simulink model "floating_2_bodies_simple"  (Simulink 6.3)
settings: Solver=ode15s  StartTime=0.0  StopTime=inf  FixedStep=0.02  RelTol=1e-3
PreLoadFcn:
  | Body_Shv_Double_066
InitFcn:
  | mech_slider_open_ShV(gcs);
libraries: mblibv1 x12
settings Model: LastModifiedBy=Alex
settings SimMechanicsCC: VisOnUpdateDiagram=on  VisDuringSimulation=on

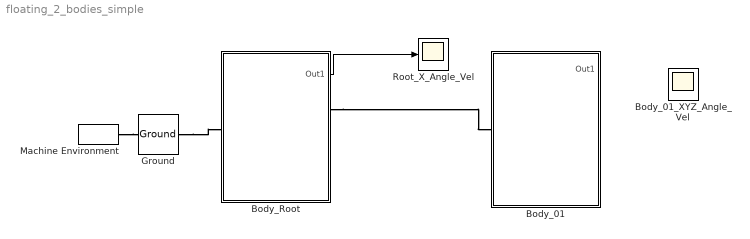
== system floating_2_bodies_simple ==
  Body_01 : Subsystem
  Body_01_XYZ_Angle_Vel : Scope
      settings: TimeRange=600  YMin=-25  YMax=2.5
  Body_Root : Subsystem
  Ground : mblibv1/Bodies/Ground  LeftPortType=env  RightPortType=workingframe  PhysicalDomain=Mechanical  DialogClass=GroundBlock  CoordPosition=[0 0 0]  CoordPositionUnits=m  StateVectorMgrId=-1  MachineId=[1 1]  ShowEnvPort=on
  Machine Environment : mblibv1/Bodies/Machine Environment  Tag=Factory ground  DialogController=MECH.DialogSource  PortType=env  PhysicalDomain=Mechanical  DialogTemplateClass=MECH.MachineEnvironment  SyncWhenCopied=off  Gravity=[0 0 0]  GravityUnits=m/s^2  GravityAsSignal=off  Dimensionality=Auto-detect  AnalysisType=Forward dynamics  LinearAssemblyTolerance=1e-3  LinearAssemblyToleranceUnits=m  AngularAssemblyTolerance=1e-3  AngularAssemblyToleranceUnits=rad  ConstraintSolverType=Stabilizing  ConstraintRelTolerance=1e-4  ConstraintAbsTolerance=1e-4  UseRobustSingularityHandling=off  StatePerturbationType=Fixed  PerturbationSize=1e-5  VisualizeMachine=on
  Root_X_Angle_Vel : Scope
      settings: TimeRange=600  YMin=-125  YMax=100
  wires:
  Body_Root/1(Out1) -> Root_X_Angle_Vel/1
  ? -> Body_01_XYZ_Angle_Vel/1
  connections:
  Machine Environment/RConn1 -- Ground/LConn1
  Ground/RConn1 -- Body_Root/LConn1
  Body_Root/RConn1 -- Body_01/LConn1

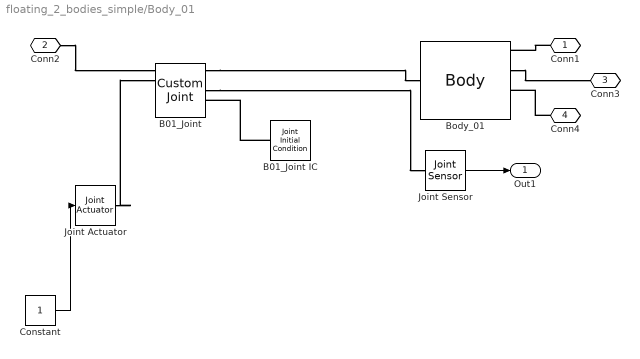
== system floating_2_bodies_simple/Body_01 ==
  B01_Joint : mblibv1/Joints/Custom Joint  PhysicalDomain=mechanical  SubClassName=custom_joint  LeftPortType=blob  RightPortType=blob  LConnTagsString=__newl0|SA1|SA2|SA3|SA4  RConnTagsString=__newr0|SA1|SA2|SA3|SA4  NumSAPorts=8  CutJoint=off  MarkAsCut=off  Primitives=revolute_revolute_revolute  PrimitiveProps=R3$WORLD$[0 0 1]$revolute#R1$WORLD$[1 0 0]$revolute#R2$WORLD$[0 1 0]$revolute  DialogClass=JointBlock
  B01_Joint IC : mblibv1/Sensors &  Actuators/Joint Initial Condition  Orientation=left  PhysicalDomain=mechanical  DialogClass=InitialConditionBlock  InitialConditions=P1$false$0$m$rad$0$m/s$rad/s#P2$false$0$m$rad$0$m/s$rad/s#P3$false$0$m$rad$0$m/s$rad/s#R1$false$0$m$rad$0$m/s$rad/s#R2$false$0$m$rad$0$m/s$rad/s#R3$false$30$m$deg$0$m/s$rad/s#S$false$0$m$rad$0$m/s$rad/s
  Body_01 : mblibv1/Bodies/Body  PhysicalDomain=mechanical  SubClassName=Unknown  LeftPortType=workingframe  RightPortType=workingframe  LConnTagsString=CS1  RConnTagsString=CS2|CS3|CS4|CS5  DialogClass=MechanicalBodyBlock  Mass=1  MassUnits=kg  InertiaUnits=kg*m^2  Inertia=[ 1/12 0 0; 0 .001 0; 0 0 1/12]  Shape=Cylinder  ShapeDims=[1 1]  ShapeUnits=m  ShapeUse=false  Density=1  DensityUnits=kg/m^3  DensityUse=false  CG=Left$CG$[0 -Body_Size 0]$CS1$CS1$m$[0 0 0]$Euler X-Y-Z$deg$WORLD$false  WorkingFrames=Left$CS1$[0 0 0]$ADJOINING$ADJOINING$m$[0 0 0]$Euler X-Y-Z$deg$WORLD$true#Right$CS2$[0 -Body_Size 0]$CG$CG$m$[0 0 0]$Euler X-Y-Z$deg$WORLD$true#Right$CS3$[-0.5*Body_Size -Body_Size 0]$CG$CG$m$[0 0 0]$Euler X-Y-Z$deg$WORLD$true#Right$CS4$[0.5*Body_Size -Body_Size 0]$CG$CG$m$[0 0 0]$Euler X-Y-Z$deg$WORLD$true#Right$CS5$[0 -Body_Size -0.2*Body_Size]$CG$CG$m$[0 0 0]$Euler X-Y-Z$deg$WORLD$true
  Constant : Constant
  Joint Actuator : mblibv1/Sensors &  Actuators/Joint Actuator  PhysicalDomain=Mechanical  PortType=blob  ActuationStyle=Force  AngleUnits=deg  ArcVelocityUnits=deg/s  ArcAccelerationUnits=deg/s^2  CoordPositionUnits=m  VelocityUnits=m/s  AccelerationUnits=m/s^2  ForceUnits=N  TorqueUnits=N-m  ActiveIO=on  Width=1  DialogClass=MechanicalActuatorBlock  Primitive=R1  ReferenceFrame=Absolute (INERTIAL)
  Joint Sensor : mblibv1/Sensors &  Actuators/Joint Sensor  PhysicalDomain=Mechanical  PortType=blob  Muxed=on  Pose=off  Angle=off  AngleUnits=deg  ArcVelocity=on  ArcVelocityUnits=deg/s  ArcAcceleration=off  ArcAccelerationUnits=deg/s^2  CoordPosition=on  CoordPositionUnits=m  Velocity=off  VelocityUnits=m/s  Acceleration=off  AccelerationUnits=m/s^2  Quaternion=on  QuaternionDT=off  QuaternionDDT=off  QuaternionUnits=off  OutputVector=[ 1 ]  ActiveIO=on  Width=1  DialogClass=MechanicalSensorBlock  Primitive=R3  Force=off  ForceUnits=N  Torque=off  TorqueUnits=N-m  ReferenceFrame=Absolute (INERTIAL)  ReactionSensedSide=Base  ReactionReferenceFrame=Local (Body CS)  ReactionForce=off  ReactionForceUnits=N  ReactionMoment=off  ReactionMomentUnits=N-m
  Conn1 : PMIOPort  Orientation=left  Port=1  Side=Right
  Conn2 : PMIOPort  Port=2  Side=Left
  Conn3 : PMIOPort  Orientation=left  Port=3  Side=Right
  Conn4 : PMIOPort  Orientation=left  Port=4  Side=Right
  Out1 : Outport
  wires:
  Joint Sensor/1 -> Out1/1
  Constant/1 -> Joint Actuator/1
  connections:
  B01_Joint/RConn1 -- Body_01/LConn1
  B01_Joint/RConn3 -- Joint Sensor/LConn1
  Conn1/RConn1 -- Body_01/RConn1
  Conn2/RConn1 -- B01_Joint/LConn1
  Conn4/RConn1 -- Body_01/RConn3
  B01_Joint IC/RConn1 -- B01_Joint/RConn4
  Body_01/RConn2 -- Conn3/RConn1
  Joint Actuator/RConn1 -- B01_Joint/LConn2

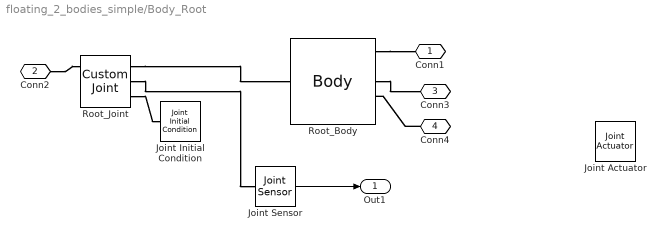
== system floating_2_bodies_simple/Body_Root ==
  Joint Actuator : mblibv1/Sensors &  Actuators/Joint Actuator  PhysicalDomain=Mechanical  PortType=blob  ActuationStyle=Force  AngleUnits=deg  ArcVelocityUnits=deg/s  ArcAccelerationUnits=deg/s^2  CoordPositionUnits=m  VelocityUnits=m/s  AccelerationUnits=m/s^2  ForceUnits=N  TorqueUnits=N-m  ActiveIO=off  Width=0  DialogClass=MechanicalActuatorBlock  Primitive=None  ReferenceFrame=Absolute (INERTIAL)
  Joint Initial Condition : mblibv1/Sensors &  Actuators/Joint Initial Condition  Orientation=left  PhysicalDomain=mechanical  DialogClass=InitialConditionBlock  InitialConditions=P1$false$0$m$rad$0$m/s$rad/s#P2$false$0$m$rad$0$m/s$rad/s#P3$false$0$m$rad$0$m/s$rad/s#R1$true$0$m$rad$1$m/s$rad/s#R2$false$0$m$rad$.0$m/s$rad/s#R3$false$0$m$rad$.5$m/s$rad/s#S$false$0$m$rad$0$m/s$rad/s
  Joint Sensor : mblibv1/Sensors &  Actuators/Joint Sensor  PhysicalDomain=Mechanical  PortType=blob  Muxed=on  Pose=off  Angle=off  AngleUnits=deg  ArcVelocity=on  ArcVelocityUnits=deg/s  ArcAcceleration=off  ArcAccelerationUnits=deg/s^2  CoordPosition=on  CoordPositionUnits=m  Velocity=off  VelocityUnits=m/s  Acceleration=off  AccelerationUnits=m/s^2  Quaternion=on  QuaternionDT=off  QuaternionDDT=off  QuaternionUnits=off  OutputVector=[ 1 ]  ActiveIO=on  Width=1  DialogClass=MechanicalSensorBlock  Primitive=R1  Force=off  ForceUnits=N  Torque=off  TorqueUnits=N-m  ReferenceFrame=Absolute (INERTIAL)  ReactionSensedSide=Base  ReactionReferenceFrame=Local (Body CS)  ReactionForce=off  ReactionForceUnits=N  ReactionMoment=off  ReactionMomentUnits=N-m
  Root_Body : mblibv1/Bodies/Body  PhysicalDomain=mechanical  SubClassName=Unknown  LeftPortType=workingframe  RightPortType=workingframe  LConnTagsString=CG  RConnTagsString=CS1|CS2|CS3|CS4|CS5  DialogClass=MechanicalBodyBlock  Mass=1  MassUnits=kg  InertiaUnits=kg*m^2  Inertia=[ 1/12 0 0; 0 .001 0; 0 0 1/12]  Shape=Cylinder  ShapeDims=[1 1]  ShapeUnits=m  ShapeUse=false  Density=1  DensityUnits=kg/m^3  DensityUse=false  CG=Left$CG$[0 0 0]$WORLD$WORLD$m$[0 0 0]$Euler X-Y-Z$deg$WORLD$true  WorkingFrames=Right$CS1$[0 Body_Size 0]$CG$CG$m$[0 0 0]$Euler X-Y-Z$deg$WORLD$true#Right$CS2$[0 -Body_Size 0]$CG$CG$m$[0 0 0]$Euler X-Y-Z$deg$WORLD$true#Right$CS3$[-0.4*Body_Size Body_Size 0]$CG$CG$m$[0 0 0]$Euler X-Y-Z$deg$WORLD$true#Right$CS4$[0.4*Body_Size Body_Size 0]$CG$CG$m$[0 0 0]$Euler X-Y-Z$deg$WORLD$true#Right$CS5$[0 Body_Size -0.2*Body_Size]$CG$CG$m$[0 0 0]$Euler X-Y-Z$deg$WORLD$true
  Root_Joint : mblibv1/Joints/Custom Joint  PhysicalDomain=mechanical  SubClassName=custom_joint  LeftPortType=blob  RightPortType=blob  LConnTagsString=__newl0|SA1|SA2  RConnTagsString=__newr0|SA1|SA2  NumSAPorts=4  CutJoint=off  MarkAsCut=off  Primitives=prismatic_prismatic_prismatic_revolute_revolute_revolute  PrimitiveProps=P1$WORLD$[1 0 0]$prismatic#P2$WORLD$[0 1 0]$prismatic#P3$WORLD$[0 0 1]$prismatic#R1$WORLD$[1 0 0]$revolute#R2$WORLD$[0 1 0]$revolute#R3$WORLD$[0 0 1]$revolute  DialogClass=JointBlock
  Conn1 : PMIOPort  Orientation=left  Port=1  Side=Right
  Conn2 : PMIOPort  Port=2  Side=Left
  Conn3 : PMIOPort  Orientation=left  Port=3  Side=Right
  Conn4 : PMIOPort  Orientation=left  Port=4  Side=Right
  Out1 : Outport
  wires:
  Joint Sensor/1 -> Out1/1
  connections:
  Root_Joint/RConn2 -- Joint Sensor/LConn1
  Conn2/RConn1 -- Root_Joint/LConn1
  Conn4/RConn1 -- Root_Body/RConn4
  Root_Body/RConn3 -- Conn3/RConn1
  Root_Joint/RConn1 -- Root_Body/LConn1
  Root_Body/RConn1 -- Conn1/RConn1
  Root_Joint/RConn3 -- Joint Initial Condition/RConn1
